simulink model "Control_model_10DOF_fin"  (R2016b)
settings: Solver=FixedStepAuto  StartTime=0.0  StopTime=10  FixedStep=0.0001  RelTol=1e-3
InitFcn:
  | Initialisation_ctr_10DOF_fin
values from neighbouring files (symbols this model uses):
  COM_Parameters = [-lpelvis/2;r2;0]    [Initialisation_ctr_10DOF_fin.m]
  DH_Parameters = [hfoot 0 ... (first row only)    [Initialisation_ctr_10DOF_fin.m]
  dTrunk = trunklbd(3)    [Initialisation_ctr_10DOF_fin.m]
  dxFootSM = dxFoot    [Initialisation_ctr_10DOF_fin.m]
  dxTrunk = 0.1    [Initialisation_ctr_10DOF_fin.m]
  Foot_Parameters = [0;-(lFoot/2-lHeel);0]    [Initialisation_ctr_10DOF_fin.m]
  HAA2HEE = [0; 0; 0.001]    [Initialisation_ctr_10DOF_fin.m]
  HEE2HFE = 0.5*[0.2; 0; 0]    [Initialisation_ctr_10DOF_fin.m]
  height_vrp = CoM_position(1)    [Initialisation_ctr_10DOF_fin.m]
  hTrunk = trunklbd(1)    [Initialisation_ctr_10DOF_fin.m]
  initial_CoM_position = R*CoM_position    [Initialisation_ctr_10DOF_fin.m]
  initial_CoM_velocity = [0;0;0]    [Initialisation_ctr_10DOF_fin.m]
  initial_left_foot = [0;0;-stance_width/2]    [Initialisation_ctr_10DOF_fin.m]
  initial_right_foot = [0;0;stance_width/2]    [Initialisation_ctr_10DOF_fin.m]
  initial_RorL = 0    [Initialisation_ctr_10DOF_fin.m]
  jointsinitial = [9;-15;6;0;0;6;-15;9]/180*pi    [Initialisation_ctr_10DOF_fin.m]
  K_DCM = 4.3*[1 0 0 ... (first row only)    [Initialisation_ctr_10DOF_fin.m]
  kD_left = mbody*[0.95 0 0 0 ... (first row only)    [Initialisation_ctr_10DOF_fin.m]
  kD_right = mbody*[0.12 0 0 0 ... (first row only)    [Initialisation_ctr_10DOF_fin.m]
  kI_left = mbody*[35 0 0 0 ... (first row only)    [Initialisation_ctr_10DOF_fin.m]
  kI_right = mbody*[38.2 0 0 0 ... (first row only)    [Initialisation_ctr_10DOF_fin.m]
  kP_left = mbody*[75 0 0 0 ... (first row only)    [Initialisation_ctr_10DOF_fin.m]
  kP_right = mbody*[5.6 0 0 0 ... (first row only)    [Initialisation_ctr_10DOF_fin.m]
  Lenght = [lShank;lThigh]    [Initialisation_ctr_10DOF_fin.m]
  lFootSM = lFoot    [Initialisation_ctr_10DOF_fin.m]
  lpelvis = wPelvis    [Initialisation_ctr_10DOF_fin.m]
  mass = mbody    (= 60)    [Initialisation_ctr_10DOF_fin.m]
  Masses = [mThigh; mShank; mTrunk]    [Initialisation_ctr_10DOF_fin.m]
  nb_step = 4    [Initialisation_ctr_10DOF_fin.m]
  nb_step_pattern = 20    [Initialisation_ctr_10DOF_fin.m]
  Pelvis_Parameters = [-lpelvis/2;hTrunk/2;0]    [Initialisation_ctr_10DOF_fin.m]
  stance_width = lpelvis    [Initialisation_ctr_10DOF_fin.m]
  stride_lenght = 0.50    (= 0.5)    [Initialisation_ctr_10DOF_fin.m]
  T_DS = time_DS    (= 0.4)    [Initialisation_ctr_10DOF_fin.m]
  T_IT = time_DS    (= 0.4)    [Initialisation_ctr_10DOF_fin.m]
  T_SS = time_swing    (= 1.6)    [Initialisation_ctr_10DOF_fin.m]
  time_DS = (time_stance-time_swing)/2    (= 0.4)    [Initialisation_ctr_10DOF_fin.m]
  time_stance = 60/100*time_stride    (= 2.4)    [Initialisation_ctr_10DOF_fin.m]
  time_step = time_stride/2    (= 2)    [Initialisation_ctr_10DOF_fin.m]
  time_swing = 40/100*time_stride    (= 1.6)    [Initialisation_ctr_10DOF_fin.m]
  validity_angle = [-20*pi/180 20*pi/180 ... (first row only)    [Initialisation_ctr_10DOF_fin.m]
  wTrunk = trunklbd(2)    [Initialisation_ctr_10DOF_fin.m]
  x4CoM = CoM_position(1)-XR4(1)    [Initialisation_ctr_10DOF_fin.m]
undefined symbols (not defined in the file or in its folder): dsegment, hFoot, l, lFoot, omega0_x, omega0_z, rho, wPelvis, X, Xp_x, Xp_z, Y, Z
undefined symbols (not defined in the file): k_grf, lShankSM, lThighSM, mShank, mThigh
libraries: nesl_utility x247, sm_lib x215, dspindex x12, FootPlacementLibrary x8, dspsigops x4, dspswit3 x1
(part 4 of 18)

== system Control_model_10DOF_fin/Time//State Machine/Step counter ==
  state : Inport
  Constant1 : Constant  Value=4
  Constant2 : Constant  Value=0
  Counter : dspswit3/Counter  Direction=Up  CountEvent=Rising edge  CounterSize=User defined  MaxCount=10000000000000000  InitialCount=0  Output=Count  HitValue=32  ResetInput=on  SamplesPerFrame=1  Ts=1  CntDtype=single  HitDtype=Logical
  Relational Operator3 : RelationalOperator  Operator===  OutDataTypeStr=boolean  RndMeth=Simplest
  Relational Operator4 : RelationalOperator  Operator===  OutDataTypeStr=boolean  RndMeth=Simplest
  nb_step : Outport
  wires:
  state/1 -> Relational Operator4/1, Relational Operator3/1
  Relational Operator4/1 -> Counter/2
  Constant2/1 -> Relational Operator4/2
  Constant1/1 -> Relational Operator3/2
  Relational Operator3/1 -> Counter/1
  Counter/1 -> nb_step/1

== system Control_model_10DOF_fin/Trajectory generator/DCM trajectory ==
  feet_positions : Inport
  time : Inport  Port=2
  State : Inport  Port=3
  DS : Subsystem  TreatAsAtomicUnit=on
  Finish_swing_phase/SS : Subsystem  TreatAsAtomicUnit=on
  Initial_Transfert : Subsystem  TreatAsAtomicUnit=on
  Merge3 : Merge  Inputs=4
  Merge4 : Merge  Inputs=4
  Stance_position : Subsystem  TreatAsAtomicUnit=on
  Switch Case : SwitchCase  CaseConditions={0,1,[2,3],4}  ShowDefaultCase=off
  DCM_position : Outport
  DCM_velocity : Outport  Port=2
  wires:
  State/1 -> Switch Case/1
  Switch Case/1 -> Stance_position/Action
  Switch Case/2 -> Initial_Transfert/Action
  Merge3/1 -> DCM_position/1
  Merge4/1 -> DCM_velocity/1
  Switch Case/3 -> Finish_swing_phase/SS/Action
  Switch Case/4 -> DS/Action
  Stance_position/1(DCM_position) -> Merge3/1
  Initial_Transfert/1(DCM_position) -> Merge3/2
  Finish_swing_phase/SS/1(DCM_position) -> Merge3/3
  DS/1(DCM_position) -> Merge3/4
  Stance_position/2(DCM_velocity) -> Merge4/1
  Initial_Transfert/2(DCM_velocity) -> Merge4/2
  Finish_swing_phase/SS/2(DCM_velocity) -> Merge4/3
  DS/2(DCM_velocity) -> Merge4/4
  Finish_swing_phase/SS/3(last_DCM_position) -> DS/1("DCM_position_ini  ")
  Finish_swing_phase/SS/4(last_DCM_velocity) -> DS/2(DCM_velocity_ini)
  feet_positions/1 -> DS/3(feet_positions), Finish_swing_phase/SS/1(feet_positions), Initial_Transfert/1(feet_positions)
  time/1 -> DS/4(time), Finish_swing_phase/SS/2(time), Initial_Transfert/2(time)

== system Control_model_10DOF_fin/Trajectory generator/Enabled and Triggered Subsystem 1 ==
  nb_step : Inport
  FK_info : Inport  Port=2
  RorL : Inport  Port=3
  State : Inport  Port=4
  Trigger : TriggerPort  VariantControl=Variant  InitialTriggerSignalState=zero
  Feet Pattern generator : Subsystem
  Merge1 : Merge  Inputs=3
  Merge2 : Merge  Inputs=3
  Mux : Mux
  Switch Case : SwitchCase  CaseConditions={[0,1],[2,3],4}  ShowDefaultCase=off
  Terminator : Terminator
  Terminator1 : Terminator
  initial position : Subsystem  TreatAsAtomicUnit=on
  initial position1 : Subsystem  TreatAsAtomicUnit=on
  initial position2 : Subsystem  TreatAsAtomicUnit=on
  selector : Subsystem
  selector1 : Subsystem
  selector2 : Subsystem
  selector3 : Subsystem
  feet_positions : Outport  PortDimensions=3*nb_step
  wires:
  nb_step/1 -> selector3/2(nb_step), selector2/2(nb_step), selector1/2(nb_step), selector/2(nb_step)
  initial position/1(initial_swing_foot) -> Merge1/1
  initial position1/1(initial_swing_foot) -> Merge1/2
  initial position/2(initial_stance_foot) -> Merge2/1
  initial position1/2(initial_stance_foot) -> Merge2/2
  Mux/1 -> feet_positions/1
  RorL/1 -> initial position2/2(RorL), initial position1/2(RorL)
  FK_info/1 -> initial position2/1(FK_info), initial position1/1(FK_info)
  selector/1(Out1) -> Mux/3
  Feet Pattern generator/1(Feet_pattern) -> selector3/1(In1), selector2/1(In1), selector1/1(In1), selector/1(In1)
  selector3/1(Out1) -> Mux/4
  Merge1/1 -> Mux/1
  Merge2/1 -> Mux/2
  State/1 -> Switch Case/1
  Switch Case/1 -> initial position/Action
  Switch Case/2 -> initial position1/Action
  Switch Case/3 -> initial position2/Action
  initial position2/1(initial_swing_foot) -> Merge1/3
  initial position2/2(initial_stance_foot) -> Merge2/3
  selector2/1(Out1) -> Terminator/1
  selector1/1(Out1) -> Terminator1/1

== system Control_model_10DOF_fin/Trajectory generator/Hip trajectory2 ==
  State : Inport
  time_Hip : Inport  Port=2
  nb_step : Inport  Port=3  PortDimensions=1
  DS : Subsystem  TreatAsAtomicUnit=on
  Finish_swing_phase : Subsystem  TreatAsAtomicUnit=on
  Initial_Transfert : Subsystem  TreatAsAtomicUnit=on
  Merge1 : Merge  Inputs=5
  SS : Subsystem  TreatAsAtomicUnit=on
  Stance_position : Subsystem  TreatAsAtomicUnit=on
  Switch Case : SwitchCase  CaseConditions={0,1,2,3,4}  ShowDefaultCase=off
  hip_trajectory : Outport
  wires:
  State/1 -> Switch Case/1
  Switch Case/1 -> Stance_position/Action
  Switch Case/2 -> Initial_Transfert/Action
  Switch Case/3 -> SS/Action
  Switch Case/4 -> Finish_swing_phase/Action
  Switch Case/5 -> DS/Action
  Stance_position/1(Hip_trajectory) -> Merge1/1
  SS/1(hip_trajectory) -> Merge1/3
  Finish_swing_phase/1(Hip_trajectory) -> Merge1/4
  DS/1(hip_trajectory) -> Merge1/5
  Merge1/1 -> hip_trajectory/1
  Initial_Transfert/1(hip_trajectory) -> Merge1/2
  time_Hip/1 -> DS/1(time_Hip), SS/1(time_Hip), Initial_Transfert/1(time_Hip)
  nb_step/1 -> SS/2(nb_step)

== system Control_model_10DOF_fin/Trajectory generator/Subsystem1 ==
  foot_position_ini : Inport  OutDataTypeStr=double  Unit=m  PortDimensions=[3 1]
  foot_position_fin : Inport  Port=2  OutDataTypeStr=double  Unit=m  PortDimensions=[3 1]
  time : Inport  Port=3  OutDataTypeStr=double  Unit=s  PortDimensions=1
  State : Inport  Port=4
  DS : Subsystem  TreatAsAtomicUnit=on
  Finish_swing_phase : Subsystem  TreatAsAtomicUnit=on
  Initial_Transfert : Subsystem  TreatAsAtomicUnit=on
  Merge1 : Merge  Inputs=5
  SS : Subsystem  TreatAsAtomicUnit=on
  Stance_position : Subsystem  TreatAsAtomicUnit=on
  Switch Case : SwitchCase  CaseConditions={0,1,2,3,4}  ShowDefaultCase=off
  swing_foot_trajectory : Outport
  wires:
  State/1 -> Switch Case/1
  Switch Case/1 -> Stance_position/Action
  Switch Case/2 -> Initial_Transfert/Action
  Switch Case/3 -> SS/Action
  Switch Case/4 -> Finish_swing_phase/Action
  Switch Case/5 -> DS/Action
  Stance_position/1(swing_foot_trajectory) -> Merge1/1
  Finish_swing_phase/1(swing_foot_trajectory) -> Merge1/4
  DS/1(swing_foot_trajectory) -> Merge1/5
  Initial_Transfert/1(swing_foot_trajectory) -> Merge1/2
  Merge1/1 -> swing_foot_trajectory/1
  SS/1(swing_foot_rajectory) -> Merge1/3
  foot_position_ini/1 -> SS/1(foot_position_ini)
  foot_position_fin/1 -> Finish_swing_phase/1(foot_position_fin), SS/2(foot_position_fin)
  time/1 -> SS/3(time_swing)

== system Control_model_10DOF_fin/Trajectory generator/knee trajectory ==
  time : Inport  OutDataTypeStr=double  Unit=s  PortDimensions=1
  State : Inport  Port=2
  joint_angle : Inport  Port=3
  RorL_phase : Inport  Port=4
  DS : Subsystem  TreatAsAtomicUnit=on
  Finish_swing_phase : Subsystem  TreatAsAtomicUnit=on
  Initial_Transfert : Subsystem  TreatAsAtomicUnit=on
  Memory : Memory
  Merge1 : Merge  Inputs=5
  Relational Operator : RelationalOperator  Operator=~=  OutDataTypeStr=boolean  RndMeth=Simplest
  SS : Subsystem  TreatAsAtomicUnit=on
  Sample and Hold : dspsigops/Sample and Hold  trig=Rising edge  initCond=0  latchinput=on
  Stance_position : Subsystem  TreatAsAtomicUnit=on
  Switch Case : SwitchCase  CaseConditions={0,1,2,3,4}  ShowDefaultCase=off
  knee_trajectory : Outport
  wires:
  State/1 -> Memory/1, Relational Operator/1, Switch Case/1
  Switch Case/1 -> Stance_position/Action
  Switch Case/2 -> Initial_Transfert/Action
  Switch Case/3 -> SS/Action
  Switch Case/4 -> Finish_swing_phase/Action
  Switch Case/5 -> DS/Action
  Stance_position/1(knee_trajectory) -> Merge1/1
  Finish_swing_phase/1(swing_trajectory) -> Merge1/4
  DS/1(knee_trajectory) -> Merge1/5
  Initial_Transfert/1(knee_trajectory) -> Merge1/2
  Merge1/1 -> knee_trajectory/1
  SS/1(knee_trajectory) -> Merge1/3
  time/1 -> DS/1(time_DS), SS/1(time_swing)
  Memory/1 -> Relational Operator/2
  Relational Operator/1 -> Sample and Hold/Trigger
  joint_angle/1 -> Sample and Hold/1
  Sample and Hold/1 -> DS/3(joint_angle), SS/3(joint_angle)
  RorL_phase/1 -> DS/2(RorL), SS/2(RorL)

== system Control_model_10DOF_fin/10DoF Walker SimMechanics Model/Foot/GRF1 Heel ==
  Conv.{,1..5} (6 alike) : nesl_utility/PS-Simulink Converter  PhysicalDomain=network_engine_domain  SubClassName=ps_output  LeftPortType=input  RightPortType=output  PseudoPeriodic=off  Frequencies=[]  Unit=1  AffineConversion=off
  External Force  and Torque : sm_lib/Forces and Torques/External Force and Torque  ForceResolutionFrame=AttachedFrame  EnableForceX=on  EnableForceY=on  EnableForceZ=on  EnableForce=off  TorqueResolutionFrame=AttachedFrame  EnableTorqueX=off  EnableTorqueY=off  EnableTorqueZ=off  EnableTorque=off
  MATLAB Function1 : MATLAB Function  TreatAsAtomicUnit=on
  Simulink-PS Converter1 : nesl_utility/Simulink-PS Converter  PhysicalDomain=network_engine_domain  SubClassName=ps_input  LeftPortType=input  RightPortType=output  PseudoPeriodic=off  Frequencies=[]  NoiseDistribution=none  NoiseParameters=[]  Unit=1  AffineConversion=off  InputFiltering=off  SimscapeFilterOrder=1  InputFilterTimeConstant=0.001  UdotUserProvided=1
  Simulink-PS Converter2 : nesl_utility/Simulink-PS Converter  PhysicalDomain=network_engine_domain  SubClassName=ps_input  LeftPortType=input  RightPortType=output  PseudoPeriodic=off  Frequencies=[]  NoiseDistribution=none  NoiseParameters=[]  Unit=1  AffineConversion=off  InputFiltering=off  SimscapeFilterOrder=1  InputFilterTimeConstant=0.001  UdotUserProvided=1
  Simulink-PS Converter3 : nesl_utility/Simulink-PS Converter  PhysicalDomain=network_engine_domain  SubClassName=ps_input  LeftPortType=input  RightPortType=output  PseudoPeriodic=off  Frequencies=[]  NoiseDistribution=none  NoiseParameters=[]  Unit=1  AffineConversion=off  InputFiltering=off  SimscapeFilterOrder=1  InputFilterTimeConstant=0.001  UdotUserProvided=1
  Transform  Sensor : sm_lib/Frames and Transforms/Transform Sensor  MeasurementFrame=World  SenseAngle=off  SenseAxis=off  SenseAngle1=off  SenseAngle2=off  SenseAngle3=off  SenseQ=off  SenseR=off  SenseOmegaX=off  SenseOmegaY=off  SenseOmegaZ=off  SenseOmega1=off  SenseOmega2=off  SenseOmega3=off  SenseQDot=off  SenseRDot=off  SenseAlphaX=off  SenseAlphaY=off  SenseAlphaZ=off  SenseAlpha1=off  SenseAlpha2=off  SenseAlpha3=off  SenseQDDot=off  SenseRDDot=off  SenseX=on  SenseY=on  SenseZ=on  SenseRad=off  SenseAzim=off  SenseDist=off  SenseInc=off  SenseXDot=on  SenseYDot=on  SenseZDot=on  SenseRadDot=off  SenseAzimDot=off  SenseDistDot=off  SenseIncDot=off  SenseXDDot=off  SenseYDDot=off  SenseZDDot=off  SenseRadDDot=off  SenseAzimDDot=off  SenseDistDDot=off  SenseIncDDot=off
  k : Constant  Value=k
  Conn2 : PMIOPort  Port=1  Side=Right
  Conn1 : PMIOPort  Port=2  Side=Left
  wires:
  Conv.5/1 -> MATLAB Function1/6(dz)
  Conv.4/1 -> MATLAB Function1/5(z)
  Conv.3/1 -> MATLAB Function1/4(dy)
  Conv./1 -> MATLAB Function1/1(x)
  Conv.2/1 -> MATLAB Function1/3(y)
  Conv.1/1 -> MATLAB Function1/2(dx)
  MATLAB Function1/3(Fz) -> Simulink-PS Converter3/1
  k/1 -> MATLAB Function1/7(k)
  MATLAB Function1/1(Fx) -> Simulink-PS Converter1/1
  MATLAB Function1/2(Fy) -> Simulink-PS Converter2/1
  connections:
  Transform  Sensor/RConn7 -- Conv.5/LConn1
  Transform  Sensor/RConn6 -- Conv.3/LConn1
  Transform  Sensor/RConn5 -- Conv.1/LConn1
  Transform  Sensor/RConn4 -- Conv.4/LConn1
  Transform  Sensor/RConn3 -- Conv.2/LConn1
  Transform  Sensor/RConn2 -- Conv./LConn1
  External Force  and Torque/LConn3 -- Simulink-PS Converter3/RConn1
  External Force  and Torque/LConn2 -- Simulink-PS Converter2/RConn1
  External Force  and Torque/LConn1 -- Simulink-PS Converter1/RConn1
  Transform  Sensor/RConn1 -- Conn1/RConn1 -- External Force  and Torque/RConn1
  Transform  Sensor/LConn1 -- Conn2/RConn1

== system Control_model_10DOF_fin/10DoF Walker SimMechanics Model/Foot/GRF1 Toe ==
  Conv.{,1..5} (6 alike) : nesl_utility/PS-Simulink Converter  PhysicalDomain=network_engine_domain  SubClassName=ps_output  LeftPortType=input  RightPortType=output  PseudoPeriodic=off  Frequencies=[]  Unit=1  AffineConversion=off
  External Force  and Torque : sm_lib/Forces and Torques/External Force and Torque  ForceResolutionFrame=AttachedFrame  EnableForceX=on  EnableForceY=on  EnableForceZ=on  EnableForce=off  TorqueResolutionFrame=AttachedFrame  EnableTorqueX=off  EnableTorqueY=off  EnableTorqueZ=off  EnableTorque=off
  MATLAB Function1 : MATLAB Function  TreatAsAtomicUnit=on
  Scope : Scope
  Simulink-PS Converter1 : nesl_utility/Simulink-PS Converter  PhysicalDomain=network_engine_domain  SubClassName=ps_input  LeftPortType=input  RightPortType=output  PseudoPeriodic=off  Frequencies=[]  NoiseDistribution=none  NoiseParameters=[]  Unit=1  AffineConversion=off  InputFiltering=off  SimscapeFilterOrder=1  InputFilterTimeConstant=0.001  UdotUserProvided=1
  Simulink-PS Converter2 : nesl_utility/Simulink-PS Converter  PhysicalDomain=network_engine_domain  SubClassName=ps_input  LeftPortType=input  RightPortType=output  PseudoPeriodic=off  Frequencies=[]  NoiseDistribution=none  NoiseParameters=[]  Unit=1  AffineConversion=off  InputFiltering=off  SimscapeFilterOrder=1  InputFilterTimeConstant=0.001  UdotUserProvided=1
  Simulink-PS Converter3 : nesl_utility/Simulink-PS Converter  PhysicalDomain=network_engine_domain  SubClassName=ps_input  LeftPortType=input  RightPortType=output  PseudoPeriodic=off  Frequencies=[]  NoiseDistribution=none  NoiseParameters=[]  Unit=1  AffineConversion=off  InputFiltering=off  SimscapeFilterOrder=1  InputFilterTimeConstant=0.001  UdotUserProvided=1
  Transform  Sensor : sm_lib/Frames and Transforms/Transform Sensor  MeasurementFrame=World  SenseAngle=off  SenseAxis=off  SenseAngle1=off  SenseAngle2=off  SenseAngle3=off  SenseQ=off  SenseR=off  SenseOmegaX=off  SenseOmegaY=off  SenseOmegaZ=off  SenseOmega1=off  SenseOmega2=off  SenseOmega3=off  SenseQDot=off  SenseRDot=off  SenseAlphaX=off  SenseAlphaY=off  SenseAlphaZ=off  SenseAlpha1=off  SenseAlpha2=off  SenseAlpha3=off  SenseQDDot=off  SenseRDDot=off  SenseX=on  SenseY=on  SenseZ=on  SenseRad=off  SenseAzim=off  SenseDist=off  SenseInc=off  SenseXDot=on  SenseYDot=on  SenseZDot=on  SenseRadDot=off  SenseAzimDot=off  SenseDistDot=off  SenseIncDot=off  SenseXDDot=off  SenseYDDot=off  SenseZDDot=off  SenseRadDDot=off  SenseAzimDDot=off  SenseDistDDot=off  SenseIncDDot=off
  k : Constant  Value=k
  Conn2 : PMIOPort  Port=1  Side=Right
  Conn1 : PMIOPort  Port=2  Side=Left
  wires:
  MATLAB Function1/2(Fy) -> Simulink-PS Converter2/1
  MATLAB Function1/1(Fx) -> Simulink-PS Converter1/1
  k/1 -> MATLAB Function1/7(k)
  MATLAB Function1/3(Fz) -> Scope/1, Simulink-PS Converter3/1
  Conv.1/1 -> MATLAB Function1/2(dx)
  Conv.2/1 -> MATLAB Function1/3(y)
  Conv./1 -> MATLAB Function1/1(x)
  Conv.3/1 -> MATLAB Function1/4(dy)
  Conv.4/1 -> MATLAB Function1/5(z)
  Conv.5/1 -> MATLAB Function1/6(dz)
  connections:
  Transform  Sensor/LConn1 -- Conn2/RConn1
  Conn1/RConn1 -- Transform  Sensor/RConn1 -- External Force  and Torque/RConn1
  External Force  and Torque/LConn1 -- Simulink-PS Converter1/RConn1
  External Force  and Torque/LConn2 -- Simulink-PS Converter2/RConn1
  External Force  and Torque/LConn3 -- Simulink-PS Converter3/RConn1
  Transform  Sensor/RConn2 -- Conv./LConn1
  Transform  Sensor/RConn3 -- Conv.2/LConn1
  Transform  Sensor/RConn4 -- Conv.4/LConn1
  Transform  Sensor/RConn5 -- Conv.1/LConn1
  Transform  Sensor/RConn6 -- Conv.3/LConn1
  Transform  Sensor/RConn7 -- Conv.5/LConn1

== system Control_model_10DOF_fin/10DoF Walker SimMechanics Model/Foot/GRF2 Heel ==
  Conv.{,1..5} (6 alike) : nesl_utility/PS-Simulink Converter  PhysicalDomain=network_engine_domain  SubClassName=ps_output  LeftPortType=input  RightPortType=output  PseudoPeriodic=off  Frequencies=[]  Unit=1  AffineConversion=off
  External Force  and Torque : sm_lib/Forces and Torques/External Force and Torque  ForceResolutionFrame=AttachedFrame  EnableForceX=on  EnableForceY=on  EnableForceZ=on  EnableForce=off  TorqueResolutionFrame=AttachedFrame  EnableTorqueX=off  EnableTorqueY=off  EnableTorqueZ=off  EnableTorque=off
  MATLAB Function1 : MATLAB Function  TreatAsAtomicUnit=on
  Simulink-PS Converter1 : nesl_utility/Simulink-PS Converter  PhysicalDomain=network_engine_domain  SubClassName=ps_input  LeftPortType=input  RightPortType=output  PseudoPeriodic=off  Frequencies=[]  NoiseDistribution=none  NoiseParameters=[]  Unit=1  AffineConversion=off  InputFiltering=off  SimscapeFilterOrder=1  InputFilterTimeConstant=0.001  UdotUserProvided=1
  Simulink-PS Converter2 : nesl_utility/Simulink-PS Converter  PhysicalDomain=network_engine_domain  SubClassName=ps_input  LeftPortType=input  RightPortType=output  PseudoPeriodic=off  Frequencies=[]  NoiseDistribution=none  NoiseParameters=[]  Unit=1  AffineConversion=off  InputFiltering=off  SimscapeFilterOrder=1  InputFilterTimeConstant=0.001  UdotUserProvided=1
  Simulink-PS Converter3 : nesl_utility/Simulink-PS Converter  PhysicalDomain=network_engine_domain  SubClassName=ps_input  LeftPortType=input  RightPortType=output  PseudoPeriodic=off  Frequencies=[]  NoiseDistribution=none  NoiseParameters=[]  Unit=1  AffineConversion=off  InputFiltering=off  SimscapeFilterOrder=1  InputFilterTimeConstant=0.001  UdotUserProvided=1
  Transform  Sensor : sm_lib/Frames and Transforms/Transform Sensor  MeasurementFrame=World  SenseAngle=off  SenseAxis=off  SenseAngle1=off  SenseAngle2=off  SenseAngle3=off  SenseQ=off  SenseR=off  SenseOmegaX=off  SenseOmegaY=off  SenseOmegaZ=off  SenseOmega1=off  SenseOmega2=off  SenseOmega3=off  SenseQDot=off  SenseRDot=off  SenseAlphaX=off  SenseAlphaY=off  SenseAlphaZ=off  SenseAlpha1=off  SenseAlpha2=off  SenseAlpha3=off  SenseQDDot=off  SenseRDDot=off  SenseX=on  SenseY=on  SenseZ=on  SenseRad=off  SenseAzim=off  SenseDist=off  SenseInc=off  SenseXDot=on  SenseYDot=on  SenseZDot=on  SenseRadDot=off  SenseAzimDot=off  SenseDistDot=off  SenseIncDot=off  SenseXDDot=off  SenseYDDot=off  SenseZDDot=off  SenseRadDDot=off  SenseAzimDDot=off  SenseDistDDot=off  SenseIncDDot=off
  k : Constant  Value=k
  Conn2 : PMIOPort  Port=1  Side=Right
  Conn1 : PMIOPort  Port=2  Side=Left
  wires:
  Conv.5/1 -> MATLAB Function1/6(dz)
  Conv.4/1 -> MATLAB Function1/5(z)
  Conv.3/1 -> MATLAB Function1/4(dy)
  Conv./1 -> MATLAB Function1/1(x)
  Conv.2/1 -> MATLAB Function1/3(y)
  Conv.1/1 -> MATLAB Function1/2(dx)
  MATLAB Function1/3(Fz) -> Simulink-PS Converter3/1
  k/1 -> MATLAB Function1/7(k)
  MATLAB Function1/1(Fx) -> Simulink-PS Converter1/1
  MATLAB Function1/2(Fy) -> Simulink-PS Converter2/1
  connections:
  Transform  Sensor/RConn7 -- Conv.5/LConn1
  Transform  Sensor/RConn6 -- Conv.3/LConn1
  Transform  Sensor/RConn5 -- Conv.1/LConn1
  Transform  Sensor/RConn4 -- Conv.4/LConn1
  Transform  Sensor/RConn3 -- Conv.2/LConn1
  Transform  Sensor/RConn2 -- Conv./LConn1
  External Force  and Torque/LConn3 -- Simulink-PS Converter3/RConn1
  External Force  and Torque/LConn2 -- Simulink-PS Converter2/RConn1
  External Force  and Torque/LConn1 -- Simulink-PS Converter1/RConn1
  Transform  Sensor/RConn1 -- Conn1/RConn1 -- External Force  and Torque/RConn1
  Transform  Sensor/LConn1 -- Conn2/RConn1

== system Control_model_10DOF_fin/10DoF Walker SimMechanics Model/Foot/GRF2 Toe ==
  Conv.{,1..5} (6 alike) : nesl_utility/PS-Simulink Converter  PhysicalDomain=network_engine_domain  SubClassName=ps_output  LeftPortType=input  RightPortType=output  PseudoPeriodic=off  Frequencies=[]  Unit=1  AffineConversion=off
  External Force  and Torque : sm_lib/Forces and Torques/External Force and Torque  ForceResolutionFrame=AttachedFrame  EnableForceX=on  EnableForceY=on  EnableForceZ=on  EnableForce=off  TorqueResolutionFrame=AttachedFrame  EnableTorqueX=off  EnableTorqueY=off  EnableTorqueZ=off  EnableTorque=off
  MATLAB Function1 : MATLAB Function  TreatAsAtomicUnit=on
  Simulink-PS Converter1 : nesl_utility/Simulink-PS Converter  PhysicalDomain=network_engine_domain  SubClassName=ps_input  LeftPortType=input  RightPortType=output  PseudoPeriodic=off  Frequencies=[]  NoiseDistribution=none  NoiseParameters=[]  Unit=1  AffineConversion=off  InputFiltering=off  SimscapeFilterOrder=1  InputFilterTimeConstant=0.001  UdotUserProvided=1
  Simulink-PS Converter2 : nesl_utility/Simulink-PS Converter  PhysicalDomain=network_engine_domain  SubClassName=ps_input  LeftPortType=input  RightPortType=output  PseudoPeriodic=off  Frequencies=[]  NoiseDistribution=none  NoiseParameters=[]  Unit=1  AffineConversion=off  InputFiltering=off  SimscapeFilterOrder=1  InputFilterTimeConstant=0.001  UdotUserProvided=1
  Simulink-PS Converter3 : nesl_utility/Simulink-PS Converter  PhysicalDomain=network_engine_domain  SubClassName=ps_input  LeftPortType=input  RightPortType=output  PseudoPeriodic=off  Frequencies=[]  NoiseDistribution=none  NoiseParameters=[]  Unit=1  AffineConversion=off  InputFiltering=off  SimscapeFilterOrder=1  InputFilterTimeConstant=0.001  UdotUserProvided=1
  Transform  Sensor : sm_lib/Frames and Transforms/Transform Sensor  MeasurementFrame=World  SenseAngle=off  SenseAxis=off  SenseAngle1=off  SenseAngle2=off  SenseAngle3=off  SenseQ=off  SenseR=off  SenseOmegaX=off  SenseOmegaY=off  SenseOmegaZ=off  SenseOmega1=off  SenseOmega2=off  SenseOmega3=off  SenseQDot=off  SenseRDot=off  SenseAlphaX=off  SenseAlphaY=off  SenseAlphaZ=off  SenseAlpha1=off  SenseAlpha2=off  SenseAlpha3=off  SenseQDDot=off  SenseRDDot=off  SenseX=on  SenseY=on  SenseZ=on  SenseRad=off  SenseAzim=off  SenseDist=off  SenseInc=off  SenseXDot=on  SenseYDot=on  SenseZDot=on  SenseRadDot=off  SenseAzimDot=off  SenseDistDot=off  SenseIncDot=off  SenseXDDot=off  SenseYDDot=off  SenseZDDot=off  SenseRadDDot=off  SenseAzimDDot=off  SenseDistDDot=off  SenseIncDDot=off
  k : Constant  Value=k
  Conn2 : PMIOPort  Port=1  Side=Right
  Conn1 : PMIOPort  Port=2  Side=Left
  wires:
  MATLAB Function1/2(Fy) -> Simulink-PS Converter2/1
  MATLAB Function1/1(Fx) -> Simulink-PS Converter1/1
  k/1 -> MATLAB Function1/7(k)
  MATLAB Function1/3(Fz) -> Simulink-PS Converter3/1
  Conv.1/1 -> MATLAB Function1/2(dx)
  Conv.2/1 -> MATLAB Function1/3(y)
  Conv./1 -> MATLAB Function1/1(x)
  Conv.3/1 -> MATLAB Function1/4(dy)
  Conv.4/1 -> MATLAB Function1/5(z)
  Conv.5/1 -> MATLAB Function1/6(dz)
  connections:
  Transform  Sensor/LConn1 -- Conn2/RConn1
  Conn1/RConn1 -- Transform  Sensor/RConn1 -- External Force  and Torque/RConn1
  External Force  and Torque/LConn1 -- Simulink-PS Converter1/RConn1
  External Force  and Torque/LConn2 -- Simulink-PS Converter2/RConn1
  External Force  and Torque/LConn3 -- Simulink-PS Converter3/RConn1
  Transform  Sensor/RConn2 -- Conv./LConn1
  Transform  Sensor/RConn3 -- Conv.2/LConn1
  Transform  Sensor/RConn4 -- Conv.4/LConn1
  Transform  Sensor/RConn5 -- Conv.1/LConn1
  Transform  Sensor/RConn6 -- Conv.3/LConn1
  Transform  Sensor/RConn7 -- Conv.5/LConn1

== system Control_model_10DOF_fin/10DoF Walker SimMechanics Model/Foot/Scope x3 ==
  Input : Inport
  Demux : Demux  Outputs=3
  Scope1 : Scope
  Scope2 : Scope
  Scope3 : Scope
  wires:
  Input/1 -> Demux/1
  Demux/2 -> Scope1/1
  Demux/3 -> Scope2/1
  Demux/1 -> Scope3/1

== system Control_model_10DOF_fin/10DoF Walker SimMechanics Model/Foot/Virtual repellent point2 ==
  Point : Inport
  Cartesian Joint : sm_lib/Joints/Cartesian Joint  SenseConstraintForce=off  SenseConstraintForceX=off  SenseConstraintForceY=off  SenseConstraintForceZ=off  SenseConstraintTorque=off  SenseConstraintTorqueX=off  SenseConstraintTorqueY=off  SenseConstraintTorqueZ=off  SenseTotalForce=off  SenseTotalForceX=off  SenseTotalForceY=off  SenseTotalForceZ=off  SenseTotalTorque=off  SenseTotalTorqueX=off  SenseTotalTorqueY=off  SenseTotalTorqueZ=off  CompositeWrenchDir=FollowerOnBase  CompositeWrenchFrame=BaseFrame  PxEquilibriumPosition=0  PxEquilibriumPositionUnits=m  PxSpringStiffness=0  PxSpringStiffnessUnits=N/m  PxDampingCoefficient=0  PxDampingCoefficientUnits=N/(m/s)  PxTorqueActuationMode=ComputedTorque  PxMotionActuationMode=InputMotion  PxSensePosition=off  PxSenseVelocity=off  PxSenseAcceleration=off  PxSenseTorqueForce=off  PxPositionTargetSpecify=on  PxPositionTargetPriority=Low  PxPositionTargetValue=0  PxPositionTargetValueUnits=m  PxVelocityTargetSpecify=off  PxVelocityTargetPriority=High  PxVelocityTargetValue=0  PxVelocityTargetValueUnits=m/s  PyEquilibriumPosition=0  PyEquilibriumPositionUnits=m  PySpringStiffness=0  PySpringStiffnessUnits=N/m  PyDampingCoefficient=0  PyDampingCoefficientUnits=N/(m/s)  PyTorqueActuationMode=ComputedTorque  PyMotionActuationMode=InputMotion  PySensePosition=off  PySenseVelocity=off  PySenseAcceleration=off  PySenseTorqueForce=off  PyPositionTargetSpecify=on  PyPositionTargetPriority=Low  PyPositionTargetValue=0  PyPositionTargetValueUnits=m  PyVelocityTargetSpecify=off  PyVelocityTargetPriority=High  PyVelocityTargetValue=0  PyVelocityTargetValueUnits=m/s  PzEquilibriumPosition=0  PzEquilibriumPositionUnits=m  PzSpringStiffness=0  PzSpringStiffnessUnits=N/m  PzDampingCoefficient=0  PzDampingCoefficientUnits=N/(m/s)  PzTorqueActuationMode=ComputedTorque  PzMotionActuationMode=InputMotion  PzSensePosition=off  PzSenseVelocity=off  PzSenseAcceleration=off  PzSenseTorqueForce=off  PzPositionTargetSpecify=on  PzPositionTargetPriority=Low  PzPositionTargetValue=0  PzPositionTargetValueUnits=m  PzVelocityTargetSpecify=off  PzVelocityTargetPriority=High  PzVelocityTargetValue=0  PzVelocityTargetValueUnits=m/s
  Demux : Demux  Outputs=3
  Graphic : sm_lib/Body Elements/Graphic  GraphicType=Marker  MarkerShape=Sphere  MarkerSize=10  GraphicVisPropType=SimpleVisualProperties  GraphicDiffuseColor=[0.0 1.0 1.0]  GraphicSpecularColor=[0.5 0.5 0.5 1.0]  GraphicAmbientColor=[0.15 0.15 0.15 1.0]  GraphicEmissiveColor=[0.0 0.0 0.0 1.0]  GraphicShininess=75  GraphicOpacity=1.0
  Memory2 : Memory  X0=[0;0;0]
  Rigid Transform1 : sm_lib/Frames and Transforms/Rigid Transform  TranslationMethod=None  TranslationStandardOffset=0  TranslationLengthUnit=m  TranslationStandardAxis=+Z  TranslationCartesianOffset=[0 0 0]  TranslationROffset=0  TranslationROffsetUnits=m  TranslationZOffset=0  TranslationZOffsetUnits=m  TranslationThetaOffset=0  TranslationThetaOffsetUnits=deg  RotationMethod=None  RotationAngleUnits=deg  RotationStandardAxis=+Z  RotationAngle=0.0  RotationArbitraryAxis=[0 0 1]  FollAlignAxisA=+X  BaseAlignAxisA=+Y  FollAlignAxisB=+Y  BaseAlignAxisB=+Z  RotationSequenceAxes=FollowerAxes  RotationSequence=XYX  RotationSequenceAngles=[0 0 0]  RotationSequenceAnglesUnits=deg  RotationMatrix=[1 0 0; 0 1 0; 0 0 1]
  Simulink-PS Converter1 : nesl_utility/Simulink-PS Converter  PhysicalDomain=network_engine_domain  SubClassName=ps_input  LeftPortType=input  RightPortType=output  PseudoPeriodic=off  Frequencies=[]  NoiseDistribution=none  NoiseParameters=[]  Unit=m  AffineConversion=on  InputFiltering=off  SimscapeFilterOrder=1  InputFilterTimeConstant=0.001  UdotUserProvided=1
  Simulink-PS Converter2 : nesl_utility/Simulink-PS Converter  PhysicalDomain=network_engine_domain  SubClassName=ps_input  LeftPortType=input  RightPortType=output  PseudoPeriodic=off  Frequencies=[]  NoiseDistribution=none  NoiseParameters=[]  Unit=m  AffineConversion=on  InputFiltering=off  SimscapeFilterOrder=1  InputFilterTimeConstant=0.001  UdotUserProvided=1
  Simulink-PS Converter7 : nesl_utility/Simulink-PS Converter  PhysicalDomain=network_engine_domain  SubClassName=ps_input  LeftPortType=input  RightPortType=output  PseudoPeriodic=off  Frequencies=[]  NoiseDistribution=none  NoiseParameters=[]  Unit=m  AffineConversion=on  InputFiltering=off  SimscapeFilterOrder=1  InputFilterTimeConstant=0.001  UdotUserProvided=1
  Sum : Sum  Inputs=|++
  Base : PMIOPort  Port=1  Side=Left
  wires:
  Demux/1 -> Simulink-PS Converter7/1
  Demux/2 -> Simulink-PS Converter1/1
  Demux/3 -> Simulink-PS Converter2/1
  Memory2/1 -> Demux/1
  Sum/1 -> Memory2/1
  Point/1 -> Sum/1
  connections:
  Rigid Transform1/LConn1 -- Cartesian Joint/RConn1
  Simulink-PS Converter7/RConn1 -- Cartesian Joint/LConn2
  Rigid Transform1/RConn1 -- Graphic/RConn1
  Simulink-PS Converter1/RConn1 -- Cartesian Joint/LConn3
  Simulink-PS Converter2/RConn1 -- Cartesian Joint/LConn4
  Base/RConn1 -- Cartesian Joint/LConn1

== system Control_model_10DOF_fin/10DoF Walker SimMechanics Model/Foot1/GRF1 Heel ==
  Conv.{,1..5} (6 alike) : nesl_utility/PS-Simulink Converter  PhysicalDomain=network_engine_domain  SubClassName=ps_output  LeftPortType=input  RightPortType=output  PseudoPeriodic=off  Frequencies=[]  Unit=1  AffineConversion=off
  External Force  and Torque : sm_lib/Forces and Torques/External Force and Torque  ForceResolutionFrame=AttachedFrame  EnableForceX=on  EnableForceY=on  EnableForceZ=on  EnableForce=off  TorqueResolutionFrame=AttachedFrame  EnableTorqueX=off  EnableTorqueY=off  EnableTorqueZ=off  EnableTorque=off
  MATLAB Function1 : MATLAB Function  TreatAsAtomicUnit=on
  Scope : Scope
  Simulink-PS Converter1 : nesl_utility/Simulink-PS Converter  PhysicalDomain=network_engine_domain  SubClassName=ps_input  LeftPortType=input  RightPortType=output  PseudoPeriodic=off  Frequencies=[]  NoiseDistribution=none  NoiseParameters=[]  Unit=1  AffineConversion=off  InputFiltering=off  SimscapeFilterOrder=1  InputFilterTimeConstant=0.001  UdotUserProvided=1
  Simulink-PS Converter2 : nesl_utility/Simulink-PS Converter  PhysicalDomain=network_engine_domain  SubClassName=ps_input  LeftPortType=input  RightPortType=output  PseudoPeriodic=off  Frequencies=[]  NoiseDistribution=none  NoiseParameters=[]  Unit=1  AffineConversion=off  InputFiltering=off  SimscapeFilterOrder=1  InputFilterTimeConstant=0.001  UdotUserProvided=1
  Simulink-PS Converter3 : nesl_utility/Simulink-PS Converter  PhysicalDomain=network_engine_domain  SubClassName=ps_input  LeftPortType=input  RightPortType=output  PseudoPeriodic=off  Frequencies=[]  NoiseDistribution=none  NoiseParameters=[]  Unit=1  AffineConversion=off  InputFiltering=off  SimscapeFilterOrder=1  InputFilterTimeConstant=0.001  UdotUserProvided=1
  Transform  Sensor : sm_lib/Frames and Transforms/Transform Sensor  MeasurementFrame=World  SenseAngle=off  SenseAxis=off  SenseAngle1=off  SenseAngle2=off  SenseAngle3=off  SenseQ=off  SenseR=off  SenseOmegaX=off  SenseOmegaY=off  SenseOmegaZ=off  SenseOmega1=off  SenseOmega2=off  SenseOmega3=off  SenseQDot=off  SenseRDot=off  SenseAlphaX=off  SenseAlphaY=off  SenseAlphaZ=off  SenseAlpha1=off  SenseAlpha2=off  SenseAlpha3=off  SenseQDDot=off  SenseRDDot=off  SenseX=on  SenseY=on  SenseZ=on  SenseRad=off  SenseAzim=off  SenseDist=off  SenseInc=off  SenseXDot=on  SenseYDot=on  SenseZDot=on  SenseRadDot=off  SenseAzimDot=off  SenseDistDot=off  SenseIncDot=off  SenseXDDot=off  SenseYDDot=off  SenseZDDot=off  SenseRadDDot=off  SenseAzimDDot=off  SenseDistDDot=off  SenseIncDDot=off
  k : Constant  Value=k
  Conn2 : PMIOPort  Port=1  Side=Right
  Conn1 : PMIOPort  Port=2  Side=Left
  wires:
  Conv.5/1 -> MATLAB Function1/6(dz)
  Conv.4/1 -> MATLAB Function1/5(z)
  Conv.3/1 -> MATLAB Function1/4(dy)
  Conv./1 -> MATLAB Function1/1(x)
  Conv.2/1 -> MATLAB Function1/3(y), Scope/1
  Conv.1/1 -> MATLAB Function1/2(dx)
  MATLAB Function1/3(Fz) -> Simulink-PS Converter3/1
  k/1 -> MATLAB Function1/7(k)
  MATLAB Function1/1(Fx) -> Simulink-PS Converter1/1
  MATLAB Function1/2(Fy) -> Simulink-PS Converter2/1
  connections:
  Transform  Sensor/RConn7 -- Conv.5/LConn1
  Transform  Sensor/RConn6 -- Conv.3/LConn1
  Transform  Sensor/RConn5 -- Conv.1/LConn1
  Transform  Sensor/RConn4 -- Conv.4/LConn1
  Transform  Sensor/RConn3 -- Conv.2/LConn1
  Transform  Sensor/RConn2 -- Conv./LConn1
  External Force  and Torque/LConn3 -- Simulink-PS Converter3/RConn1
  External Force  and Torque/LConn2 -- Simulink-PS Converter2/RConn1
  External Force  and Torque/LConn1 -- Simulink-PS Converter1/RConn1
  Transform  Sensor/RConn1 -- Conn1/RConn1 -- External Force  and Torque/RConn1
  Transform  Sensor/LConn1 -- Conn2/RConn1

== system Control_model_10DOF_fin/10DoF Walker SimMechanics Model/Foot1/GRF1 Toe ==
  Conv.{,1..5} (6 alike) : nesl_utility/PS-Simulink Converter  PhysicalDomain=network_engine_domain  SubClassName=ps_output  LeftPortType=input  RightPortType=output  PseudoPeriodic=off  Frequencies=[]  Unit=1  AffineConversion=off
  External Force  and Torque : sm_lib/Forces and Torques/External Force and Torque  ForceResolutionFrame=AttachedFrame  EnableForceX=on  EnableForceY=on  EnableForceZ=on  EnableForce=off  TorqueResolutionFrame=AttachedFrame  EnableTorqueX=off  EnableTorqueY=off  EnableTorqueZ=off  EnableTorque=off
  MATLAB Function1 : MATLAB Function  TreatAsAtomicUnit=on
  Scope : Scope
  Simulink-PS Converter1 : nesl_utility/Simulink-PS Converter  PhysicalDomain=network_engine_domain  SubClassName=ps_input  LeftPortType=input  RightPortType=output  PseudoPeriodic=off  Frequencies=[]  NoiseDistribution=none  NoiseParameters=[]  Unit=1  AffineConversion=off  InputFiltering=off  SimscapeFilterOrder=1  InputFilterTimeConstant=0.001  UdotUserProvided=1
  Simulink-PS Converter2 : nesl_utility/Simulink-PS Converter  PhysicalDomain=network_engine_domain  SubClassName=ps_input  LeftPortType=input  RightPortType=output  PseudoPeriodic=off  Frequencies=[]  NoiseDistribution=none  NoiseParameters=[]  Unit=1  AffineConversion=off  InputFiltering=off  SimscapeFilterOrder=1  InputFilterTimeConstant=0.001  UdotUserProvided=1
  Simulink-PS Converter3 : nesl_utility/Simulink-PS Converter  PhysicalDomain=network_engine_domain  SubClassName=ps_input  LeftPortType=input  RightPortType=output  PseudoPeriodic=off  Frequencies=[]  NoiseDistribution=none  NoiseParameters=[]  Unit=1  AffineConversion=off  InputFiltering=off  SimscapeFilterOrder=1  InputFilterTimeConstant=0.001  UdotUserProvided=1
  Transform  Sensor : sm_lib/Frames and Transforms/Transform Sensor  MeasurementFrame=World  SenseAngle=off  SenseAxis=off  SenseAngle1=off  SenseAngle2=off  SenseAngle3=off  SenseQ=off  SenseR=off  SenseOmegaX=off  SenseOmegaY=off  SenseOmegaZ=off  SenseOmega1=off  SenseOmega2=off  SenseOmega3=off  SenseQDot=off  SenseRDot=off  SenseAlphaX=off  SenseAlphaY=off  SenseAlphaZ=off  SenseAlpha1=off  SenseAlpha2=off  SenseAlpha3=off  SenseQDDot=off  SenseRDDot=off  SenseX=on  SenseY=on  SenseZ=on  SenseRad=off  SenseAzim=off  SenseDist=off  SenseInc=off  SenseXDot=on  SenseYDot=on  SenseZDot=on  SenseRadDot=off  SenseAzimDot=off  SenseDistDot=off  SenseIncDot=off  SenseXDDot=off  SenseYDDot=off  SenseZDDot=off  SenseRadDDot=off  SenseAzimDDot=off  SenseDistDDot=off  SenseIncDDot=off
  k : Constant  Value=k
  Conn2 : PMIOPort  Port=1  Side=Right
  Conn1 : PMIOPort  Port=2  Side=Left
  wires:
  MATLAB Function1/2(Fy) -> Simulink-PS Converter2/1
  MATLAB Function1/1(Fx) -> Simulink-PS Converter1/1
  k/1 -> MATLAB Function1/7(k)
  MATLAB Function1/3(Fz) -> Simulink-PS Converter3/1
  Conv.1/1 -> MATLAB Function1/2(dx)
  Conv.2/1 -> Scope/1, MATLAB Function1/3(y)
  Conv./1 -> MATLAB Function1/1(x)
  Conv.3/1 -> MATLAB Function1/4(dy)
  Conv.4/1 -> MATLAB Function1/5(z)
  Conv.5/1 -> MATLAB Function1/6(dz)
  connections:
  Transform  Sensor/LConn1 -- Conn2/RConn1
  Conn1/RConn1 -- Transform  Sensor/RConn1 -- External Force  and Torque/RConn1
  External Force  and Torque/LConn1 -- Simulink-PS Converter1/RConn1
  External Force  and Torque/LConn2 -- Simulink-PS Converter2/RConn1
  External Force  and Torque/LConn3 -- Simulink-PS Converter3/RConn1
  Transform  Sensor/RConn2 -- Conv./LConn1
  Transform  Sensor/RConn3 -- Conv.2/LConn1
  Transform  Sensor/RConn4 -- Conv.4/LConn1
  Transform  Sensor/RConn5 -- Conv.1/LConn1
  Transform  Sensor/RConn6 -- Conv.3/LConn1
  Transform  Sensor/RConn7 -- Conv.5/LConn1

== system Control_model_10DOF_fin/10DoF Walker SimMechanics Model/Foot1/GRF2 Heel ==
  Conv.{,1..5} (6 alike) : nesl_utility/PS-Simulink Converter  PhysicalDomain=network_engine_domain  SubClassName=ps_output  LeftPortType=input  RightPortType=output  PseudoPeriodic=off  Frequencies=[]  Unit=1  AffineConversion=off
  External Force  and Torque : sm_lib/Forces and Torques/External Force and Torque  ForceResolutionFrame=AttachedFrame  EnableForceX=on  EnableForceY=on  EnableForceZ=on  EnableForce=off  TorqueResolutionFrame=AttachedFrame  EnableTorqueX=off  EnableTorqueY=off  EnableTorqueZ=off  EnableTorque=off
  MATLAB Function1 : MATLAB Function  TreatAsAtomicUnit=on
  Scope : Scope
  Simulink-PS Converter1 : nesl_utility/Simulink-PS Converter  PhysicalDomain=network_engine_domain  SubClassName=ps_input  LeftPortType=input  RightPortType=output  PseudoPeriodic=off  Frequencies=[]  NoiseDistribution=none  NoiseParameters=[]  Unit=1  AffineConversion=off  InputFiltering=off  SimscapeFilterOrder=1  InputFilterTimeConstant=0.001  UdotUserProvided=1
  Simulink-PS Converter2 : nesl_utility/Simulink-PS Converter  PhysicalDomain=network_engine_domain  SubClassName=ps_input  LeftPortType=input  RightPortType=output  PseudoPeriodic=off  Frequencies=[]  NoiseDistribution=none  NoiseParameters=[]  Unit=1  AffineConversion=off  InputFiltering=off  SimscapeFilterOrder=1  InputFilterTimeConstant=0.001  UdotUserProvided=1
  Simulink-PS Converter3 : nesl_utility/Simulink-PS Converter  PhysicalDomain=network_engine_domain  SubClassName=ps_input  LeftPortType=input  RightPortType=output  PseudoPeriodic=off  Frequencies=[]  NoiseDistribution=none  NoiseParameters=[]  Unit=1  AffineConversion=off  InputFiltering=off  SimscapeFilterOrder=1  InputFilterTimeConstant=0.001  UdotUserProvided=1
  Transform  Sensor : sm_lib/Frames and Transforms/Transform Sensor  MeasurementFrame=World  SenseAngle=off  SenseAxis=off  SenseAngle1=off  SenseAngle2=off  SenseAngle3=off  SenseQ=off  SenseR=off  SenseOmegaX=off  SenseOmegaY=off  SenseOmegaZ=off  SenseOmega1=off  SenseOmega2=off  SenseOmega3=off  SenseQDot=off  SenseRDot=off  SenseAlphaX=off  SenseAlphaY=off  SenseAlphaZ=off  SenseAlpha1=off  SenseAlpha2=off  SenseAlpha3=off  SenseQDDot=off  SenseRDDot=off  SenseX=on  SenseY=on  SenseZ=on  SenseRad=off  SenseAzim=off  SenseDist=off  SenseInc=off  SenseXDot=on  SenseYDot=on  SenseZDot=on  SenseRadDot=off  SenseAzimDot=off  SenseDistDot=off  SenseIncDot=off  SenseXDDot=off  SenseYDDot=off  SenseZDDot=off  SenseRadDDot=off  SenseAzimDDot=off  SenseDistDDot=off  SenseIncDDot=off
  k : Constant  Value=k
  Conn2 : PMIOPort  Port=1  Side=Right
  Conn1 : PMIOPort  Port=2  Side=Left
  wires:
  Conv.5/1 -> MATLAB Function1/6(dz)
  Conv.4/1 -> MATLAB Function1/5(z)
  Conv.3/1 -> MATLAB Function1/4(dy)
  Conv./1 -> MATLAB Function1/1(x)
  Conv.2/1 -> Scope/1, MATLAB Function1/3(y)
  Conv.1/1 -> MATLAB Function1/2(dx)
  MATLAB Function1/3(Fz) -> Simulink-PS Converter3/1
  k/1 -> MATLAB Function1/7(k)
  MATLAB Function1/1(Fx) -> Simulink-PS Converter1/1
  MATLAB Function1/2(Fy) -> Simulink-PS Converter2/1
  connections:
  Transform  Sensor/RConn7 -- Conv.5/LConn1
  Transform  Sensor/RConn6 -- Conv.3/LConn1
  Transform  Sensor/RConn5 -- Conv.1/LConn1
  Transform  Sensor/RConn4 -- Conv.4/LConn1
  Transform  Sensor/RConn3 -- Conv.2/LConn1
  Transform  Sensor/RConn2 -- Conv./LConn1
  External Force  and Torque/LConn3 -- Simulink-PS Converter3/RConn1
  External Force  and Torque/LConn2 -- Simulink-PS Converter2/RConn1
  External Force  and Torque/LConn1 -- Simulink-PS Converter1/RConn1
  Transform  Sensor/RConn1 -- Conn1/RConn1 -- External Force  and Torque/RConn1
  Transform  Sensor/LConn1 -- Conn2/RConn1

== system Control_model_10DOF_fin/10DoF Walker SimMechanics Model/Foot1/GRF2 Toe ==
  Conv.{,1..5} (6 alike) : nesl_utility/PS-Simulink Converter  PhysicalDomain=network_engine_domain  SubClassName=ps_output  LeftPortType=input  RightPortType=output  PseudoPeriodic=off  Frequencies=[]  Unit=1  AffineConversion=off
  External Force  and Torque : sm_lib/Forces and Torques/External Force and Torque  ForceResolutionFrame=AttachedFrame  EnableForceX=on  EnableForceY=on  EnableForceZ=on  EnableForce=off  TorqueResolutionFrame=AttachedFrame  EnableTorqueX=off  EnableTorqueY=off  EnableTorqueZ=off  EnableTorque=off
  MATLAB Function1 : MATLAB Function  TreatAsAtomicUnit=on
  Scope : Scope
  Simulink-PS Converter1 : nesl_utility/Simulink-PS Converter  PhysicalDomain=network_engine_domain  SubClassName=ps_input  LeftPortType=input  RightPortType=output  PseudoPeriodic=off  Frequencies=[]  NoiseDistribution=none  NoiseParameters=[]  Unit=1  AffineConversion=off  InputFiltering=off  SimscapeFilterOrder=1  InputFilterTimeConstant=0.001  UdotUserProvided=1
  Simulink-PS Converter2 : nesl_utility/Simulink-PS Converter  PhysicalDomain=network_engine_domain  SubClassName=ps_input  LeftPortType=input  RightPortType=output  PseudoPeriodic=off  Frequencies=[]  NoiseDistribution=none  NoiseParameters=[]  Unit=1  AffineConversion=off  InputFiltering=off  SimscapeFilterOrder=1  InputFilterTimeConstant=0.001  UdotUserProvided=1
  Simulink-PS Converter3 : nesl_utility/Simulink-PS Converter  PhysicalDomain=network_engine_domain  SubClassName=ps_input  LeftPortType=input  RightPortType=output  PseudoPeriodic=off  Frequencies=[]  NoiseDistribution=none  NoiseParameters=[]  Unit=1  AffineConversion=off  InputFiltering=off  SimscapeFilterOrder=1  InputFilterTimeConstant=0.001  UdotUserProvided=1
  Transform  Sensor : sm_lib/Frames and Transforms/Transform Sensor  MeasurementFrame=World  SenseAngle=off  SenseAxis=off  SenseAngle1=off  SenseAngle2=off  SenseAngle3=off  SenseQ=off  SenseR=off  SenseOmegaX=off  SenseOmegaY=off  SenseOmegaZ=off  SenseOmega1=off  SenseOmega2=off  SenseOmega3=off  SenseQDot=off  SenseRDot=off  SenseAlphaX=off  SenseAlphaY=off  SenseAlphaZ=off  SenseAlpha1=off  SenseAlpha2=off  SenseAlpha3=off  SenseQDDot=off  SenseRDDot=off  SenseX=on  SenseY=on  SenseZ=on  SenseRad=off  SenseAzim=off  SenseDist=off  SenseInc=off  SenseXDot=on  SenseYDot=on  SenseZDot=on  SenseRadDot=off  SenseAzimDot=off  SenseDistDot=off  SenseIncDot=off  SenseXDDot=off  SenseYDDot=off  SenseZDDot=off  SenseRadDDot=off  SenseAzimDDot=off  SenseDistDDot=off  SenseIncDDot=off
  k : Constant  Value=k
  Conn2 : PMIOPort  Port=1  Side=Right
  Conn1 : PMIOPort  Port=2  Side=Left
  wires:
  MATLAB Function1/2(Fy) -> Simulink-PS Converter2/1
  MATLAB Function1/1(Fx) -> Simulink-PS Converter1/1
  k/1 -> MATLAB Function1/7(k)
  MATLAB Function1/3(Fz) -> Simulink-PS Converter3/1
  Conv.1/1 -> MATLAB Function1/2(dx)
  Conv.2/1 -> Scope/1, MATLAB Function1/3(y)
  Conv./1 -> MATLAB Function1/1(x)
  Conv.3/1 -> MATLAB Function1/4(dy)
  Conv.4/1 -> MATLAB Function1/5(z)
  Conv.5/1 -> MATLAB Function1/6(dz)
  connections:
  Transform  Sensor/LConn1 -- Conn2/RConn1
  Conn1/RConn1 -- Transform  Sensor/RConn1 -- External Force  and Torque/RConn1
  External Force  and Torque/LConn1 -- Simulink-PS Converter1/RConn1
  External Force  and Torque/LConn2 -- Simulink-PS Converter2/RConn1
  External Force  and Torque/LConn3 -- Simulink-PS Converter3/RConn1
  Transform  Sensor/RConn2 -- Conv./LConn1
  Transform  Sensor/RConn3 -- Conv.2/LConn1
  Transform  Sensor/RConn4 -- Conv.4/LConn1
  Transform  Sensor/RConn5 -- Conv.1/LConn1
  Transform  Sensor/RConn6 -- Conv.3/LConn1
  Transform  Sensor/RConn7 -- Conv.5/LConn1
